simulink model "otherformSimulink"  (R2021b)
settings: Solver=VariableStepAuto  StartTime=0.0  StopTime=5  RelTol=1e-3
values from neighbouring files (symbols this model uses):
  A_numerical = double(subs(A_linear,[x1,x1_dot,a1,a1_dot,y1,y1_dot,b1,b1_dot],[0,0,0,0,0,0,0,0]))    [Specific_Frequency_Q7.m]
  B = [0, 0; 0, 0; 0, 0; 1, 0; 0, 0; 0, 0; 0, 0; 0, 1]    [Specific_Frequency_Q7.m]
  C = [1, 0, 0, 0, 0, 0, 0, 0; 0, 0, 0, 0, 1, 0, 0, 0]    [Specific_Frequency_Q7.m]
undefined symbols (not defined in the file or in its folder): D_numerical
settings Model: Creator=ComputerMoalem  LastModifiedBy=sadeg
settings DebuggingCC: UnconnectedInputMsg=none  UnconnectedOutputMsg=none  UnconnectedLineMsg=none
settings ModelReferenceCC: EnableRefExpFcnMdlSchedulingChecks=off
settings RTWCC: DLArmComputeVersion=20.02.1

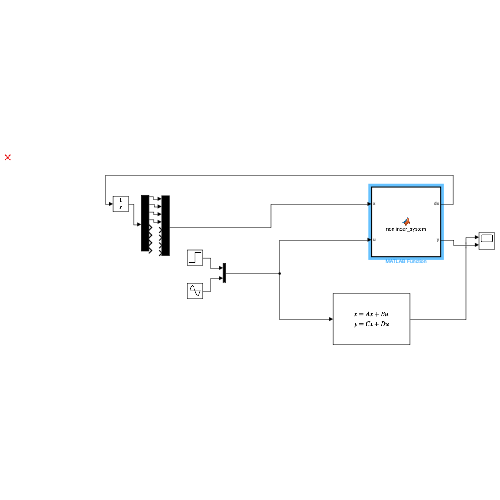
[thumbnail: Simulink's stored preview of the top-level diagram]
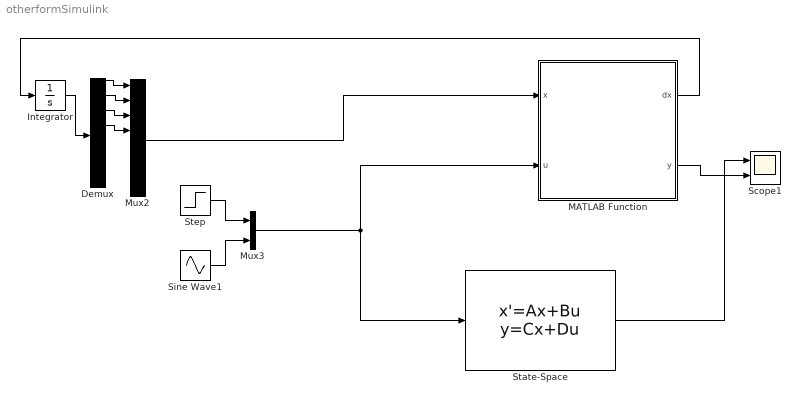
== system otherformSimulink ==
  Demux : Demux  Outputs=8
  Integrator : Integrator  InitialCondition=zeros(8,1)
  MATLAB Function : MATLAB Function  TreatAsAtomicUnit=on
  Mux2 : Mux  Inputs=8
  Mux3 : Mux  Inputs=2
  Scope1 : Scope  NumInputPorts=2
  Sine Wave1 : Sin  Frequency=4  SampleTime=0
  State-Space : StateSpace  A=A_numerical  B=B  C=C  D=D_numerical  InitialCondition=0
  Step : Step  SampleTime=0
  wires:
  State-Space/1 -> Scope1/1
  MATLAB Function/1(dx) -> Integrator/1
  Integrator/1 -> Demux/1
  Demux/1 -> Mux2/1
  Demux/2 -> Mux2/2
  Demux/3 -> Mux2/3
  Demux/4 -> Mux2/4
  ? -> ?
  ? -> ?
  ? -> ?
  ? -> ?
  Mux2/1 -> MATLAB Function/1(x)
  MATLAB Function/2(y) -> Scope1/2
  Step/1 -> Mux3/1
  Sine Wave1/1 -> Mux3/2
  Mux3/1 -> MATLAB Function/2(u), State-Space/1

== matlab function otherformSimulink/MATLAB Function ==
  data: x input size=8; u input size=2; dx output size=8; y output size=2
function [dx, y] = nonlinear_system(x, u)

    x = reshape(x, [], 1);
    assert(length(x) == 8, 'Input x must be a vector of size 8.');


    mb = 0.11;  % mass of ball (kg)
    Jb = 1.76e-5;  % rotational moment of inertia of the ball (kgm^2)
    Rb = 0.02;  % radius of the ball (m)
    g = 9.8;  % acceleration due to gravity (m/s^2)

    % B_parameter
    B_parameter = mb / (mb + (Jb / Rb^2));

    B = [0, 0; 
         0, 0; 
         0, 0; 
         1, 0; 
         0, 0; 
         0, 0; 
         0, 0; 
         0, 1];  % 8x2 matrix

    % Nonlinear dynamics equations
    dx1 = x(2);
    dx2 = B_parameter * (x(1) * x(4)^2 + x(4) * x(5) * x(8) - g * sin(x(3))) %+ B(4, :) * u;  % Input influence on dx2
    dx3 = x(4);
    dx4 = 0;

    dx5 = x(6);
    dx6 = B_parameter * (x(5) * x(8)^2 + x(1) * x(4) * x(8) - g * sin(x(7))) %+ B(8, :) * u;  % Input influence on dx6
    dx7 = x(8);
    dx8 = 0;

    % State derivative
    dx = [dx1; dx2; dx3; dx4; dx5; dx6; dx7; dx8]+ B*u;

    % Output equation: y = C*x
    C = [1, 0, 0, 0, 0, 0, 0, 0; 
         0, 0, 0, 0, 1, 0, 0, 0];  % C matrix (2x8)

    y = C * x;  % Compute the outputs
end
